simulink model "costas_pYll_qpsk_3"  (Simulink 7.1)
settings: Solver=VariableStepDiscrete  StartTime=0.0  StopTime=inf  RelTol=1e-3
libraries: dsparch4 x3, commrandsrc2 x2, simulink x2, dspsrcs4 x2, commsynccomp2 x2, commutil2 x2, commchan3 x1
settings Model: Creator=Lekha1  LastModifiedBy=Lekha1

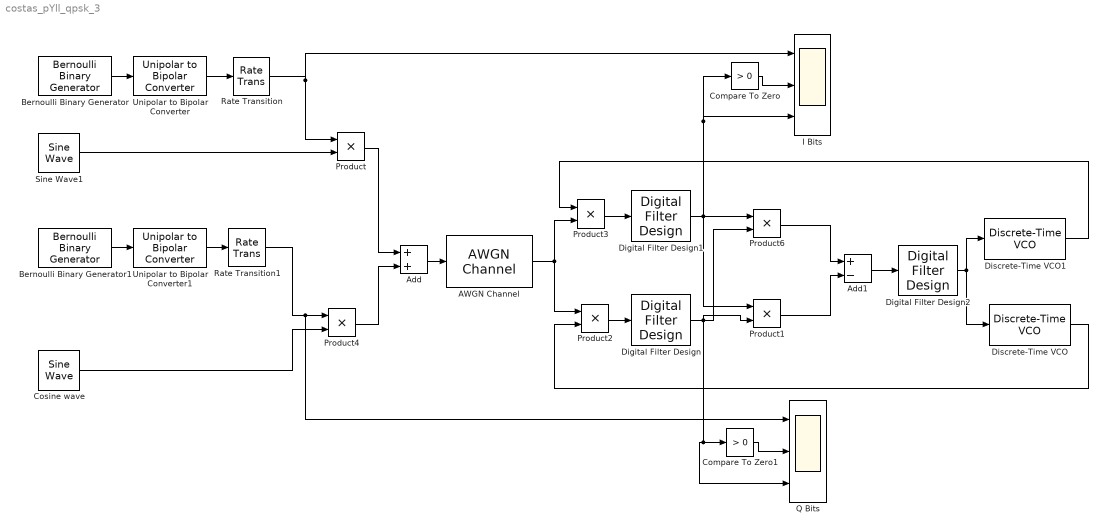
== system costas_pYll_qpsk_3 ==
  AWGN Channel : commchan3/AWGN Channel  SystemSampleTime=-1  seed=67  noiseMode="Signal to noise ratio  (SNR)"  EbNodB=10  EsNodB=10  SNRdB=5  bitsPerSym=1  Ps=1  Tsym=1  variance=1
  Add : Sum  OutDataType=sfix(16)  OutScaling=2^-10
  Add1 : Sum  Inputs=+-  OutDataType=sfix(16)  OutScaling=2^-10
  Bernoulli Binary Generator : commrandsrc2/Bernoulli Binary Generator  DialogController=commDDGCreate  DialogControllerArgs=DataTag0  SystemSampleTime=-1  P=0.5  seed=61  Ts=1/200  frameBased=off  sampPerFrame=1  orient=off  outDataType=double
  Bernoulli Binary Generator1 : commrandsrc2/Bernoulli Binary Generator  DialogController=commDDGCreate  DialogControllerArgs=DataTag1  SystemSampleTime=-1  P=0.5  seed=87  Ts=1/200  frameBased=off  sampPerFrame=1  orient=off  outDataType=double
  Compare To Zero : simulink/Logic and Bit Operations/Compare To Zero  SystemSampleTime=-1  relop=>  LogicOutDataTypeMode=uint8  ZeroCross=off
  Compare To Zero1 : simulink/Logic and Bit Operations/Compare To Zero  SystemSampleTime=-1  relop=>  LogicOutDataTypeMode=uint8  ZeroCross=off
  Cosine wave : dspsrcs4/Sine Wave  Amplitude=1  Frequency=2e3  Phase=pi/2  SampleMode=Discrete  OutComplex=Real  CompMethod=Trigonometric fcn  TableSize=Speed  SampleTime=1/(16*2e3)  SamplesPerFrame=1  dataType=double  wordLen=16  udDataType=sfix(16)  fracBitsMode=Best precision  numFracBits=15  ResetState=Restart at time zero
  Digital Filter Design : dsparch4/Digital Filter Design  SystemSampleTime=-1  mwdsp_browser_bugfix_var=off
  Digital Filter Design1 : dsparch4/Digital Filter Design  SystemSampleTime=-1  mwdsp_browser_bugfix_var=off
  Digital Filter Design2 : dsparch4/Digital Filter Design  SystemSampleTime=-1  mwdsp_browser_bugfix_var=off
  Discrete-Time VCO : commsynccomp2/Discrete-Time VCO  SystemSampleTime=-1  Ac=1  Fc=1e3  Kc=1e2  Ph=0  ts=1/16e3
  Discrete-Time VCO1 : commsynccomp2/Discrete-Time VCO  SystemSampleTime=-1  Ac=1  Fc=1e3  Kc=1e2  Ph=pi/2  ts=1/16e3
  I Bits : Scope  NumInputPorts=3
      settings: TimeRange=0.1799999999999997  YMin=-1~0~-1  YMax=1~1~1.25
  Product{,1..4,6} (6 alike) : Product  OutDataType=sfix(16)  OutScaling=2^0  RndMeth=Zero
  Q Bits : Scope  NumInputPorts=3
      settings: TimeRange=0.5  YMin=-1~0~-1  YMax=1~1~1.25
  Rate Transition : RateTransition
  Rate Transition1 : RateTransition
  Sine Wave1 : dspsrcs4/Sine Wave  Amplitude=1  Frequency=2e3  Phase=0  SampleMode=Discrete  OutComplex=Real  CompMethod=Trigonometric fcn  TableSize=Speed  SampleTime=1/(16*2e3)  SamplesPerFrame=1  dataType=double  wordLen=16  udDataType=sfix(16)  fracBitsMode=Best precision  numFracBits=15  ResetState=Restart at time zero
  Unipolar to Bipolar Converter : commutil2/Unipolar to Bipolar Converter  SystemSampleTime=-1  M=2  polarity=Positive  dataType=Same as input
  Unipolar to Bipolar Converter1 : commutil2/Unipolar to Bipolar Converter  SystemSampleTime=-1  M=2  polarity=Positive  dataType=Same as input
  wires:
  Digital Filter Design1/1 -> Compare To Zero/1, I Bits/3, Product6/1, Product1/1
  Digital Filter Design/1 -> Q Bits/3, Compare To Zero1/1, Product1/2, Product6/2
  Digital Filter Design2/1 -> Discrete-Time VCO1/1, Discrete-Time VCO/1
  Product2/1 -> Digital Filter Design/1
  Product3/1 -> Digital Filter Design1/1
  Discrete-Time VCO/1 -> Product2/2
  Rate Transition/1 -> Product/1, I Bits/1
  Bernoulli Binary Generator/1 -> Unipolar to Bipolar Converter/1
  Unipolar to Bipolar Converter/1 -> Rate Transition/1
  Sine Wave1/1 -> Product/2
  AWGN Channel/1 -> Product3/2, Product2/1
  Bernoulli Binary Generator1/1 -> Unipolar to Bipolar Converter1/1
  Unipolar to Bipolar Converter1/1 -> Rate Transition1/1
  Rate Transition1/1 -> Product4/1, Q Bits/1
  Cosine wave/1 -> Product4/2
  Product/1 -> Add/1
  Product4/1 -> Add/2
  Add/1 -> AWGN Channel/1
  Discrete-Time VCO1/1 -> Product3/1
  Compare To Zero/1 -> I Bits/2
  Compare To Zero1/1 -> Q Bits/2
  Product6/1 -> Add1/1
  Product1/1 -> Add1/2
  Add1/1 -> Digital Filter Design2/1
